simulink model "EcoSIM3_P2_C2_WIP"  (R2014b)
settings: Solver=ode1  SolverMode=SingleTasking  StartTime=0.0  StopTime=4  FixedStep=0.01  RelTol=1e-3
PostLoadFcn:
  | %, if any(exist('dsrtsu_mdlpostloadfcn', 'file') == [2, 3, 6]), try dsrtsu_mdlpostloadfcn('Execute', bdroot); catch fprintf('Error in PostLoadFcn (dsrtsu_mdlpostloadfcn) for model "%s":\n %s\n', bdroot, lasterr); end, end,
InitFcn:
  | tic
  | %Startup_EcoSIM
undefined symbols (not defined in the file or in its folder): canChannel, Controls, DriveCycles, Driver, EM_EFF_MAP, EM_PwrLoss_MAP, EngPwr, EngSpd, EngTrq, Glbl, Overwritten_Mode, Plants, Power, sigbuilder_block, Torque, Trialmap, Veh_Dynamics
libraries: simulink x135, canmsglib x113, fl_lib x104, canlib x89, nesl_utility x56, sdl_lib x29, dspsigops x6, dspswit3 x5, dspstat3 x2, commnoisgen2 x1, dspfdesign x1
(part 12 of 21)

== system EcoSIM3_P2_C2_WIP/Powertrain/Soft_ECUs_IO/VNT Vector/CANTx/EM ==
  EM : Inport
  CAN Transmit1 : canlib/CAN Transmit  BlockHandle=11751.0004  DeviceMenu=Vector Virtual 1 (Channel 2)  Device=Vector Virtual 1 (Channel 2)  ObjConstructor=canChannel('Vector', 'Virtual 1', 2)  EnablePeriodicTransmit=off  MessagePeriod=1.000
  M160_Temperature_Set_1 : Subsystem
  M161_Temperature_Set_2 : Subsystem
  M162_Temperature_Set_3 : Subsystem
  M165_Motor_Position_Info : Subsystem
  M170_Internal_States : Subsystem
  M171_Fault_Codes : Subsystem
  M172_Torque_And_Timer_Info : Subsystem
  Mux : Mux  Inputs=7
  wires:
  EM/1 -> M160_Temperature_Set_1/1(EM), M161_Temperature_Set_2/1(EM), M162_Temperature_Set_3/1(EM), M170_Internal_States/1(EM), M172_Torque_And_Timer_Info/1(EM), M165_Motor_Position_Info/1(EM), M171_Fault_Codes/1(EM)
  M165_Motor_Position_Info/1(Out1) -> Mux/1
  M172_Torque_And_Timer_Info/1(Out1) -> Mux/2
  M170_Internal_States/1(Out1) -> Mux/3
  M171_Fault_Codes/1(Out1) -> Mux/4
  M160_Temperature_Set_1/1(Out1) -> Mux/5
  M161_Temperature_Set_2/1(Out1) -> Mux/6
  M162_Temperature_Set_3/1(Out1) -> Mux/7
  Mux/1 -> CAN Transmit1/1

== system EcoSIM3_P2_C2_WIP/Powertrain/Soft_ECUs_IO/VNT Vector/CANTx/ESS ==
  ESS : Inport
  BCM_Data : Subsystem
  BCM_Limits : Subsystem
  BCM_Status : Subsystem
  wires:
  ESS/1 -> BCM_Data/1(ESS), BCM_Status/1(ESS), BCM_Limits/1(ESS)

== system EcoSIM3_P2_C2_WIP/Powertrain/Soft_ECUs_IO/VNT Vector/CANTx/Engine ==
  ICE : Inport
  Bus Selector1 : BusSelector  OutputSignals=ICE_Torque.ICE_Torque_Cmd_Nm
  CAN Pack : canmsglib/CAN Pack  CANdbFile=C:\Users\EcoCAR_HIL\Documents\Khanna\EcoSIM3_P1_0_PHEV_TCU\Final_DBC\Engine_Transmission_BAS.dbc  MsgList=ECO_Engine_MSG104  MsgName=ECO_Engine_MSG104  MsgIDType=Standard (11-bit identifier)  MsgIdentifier=104  MsgLength=2  SignalInfo=ICE_Torque_Cmd_Nm$9$15$2$2$1$0$1.000000e-02$0$0$3.276700e+02$#  NSignals=1  StartBits=str2num('[int32(9)]')  SignalSizes=str2num('[int32(15)]')  ByteOrders=str2num('[int32(2)]')  DataTypes=str2num('[int32(2)]')  MultiplexTypes=str2num('[int32(1)]')  MultiplexValues=str2num('[double(0)]')  Factors=str2num('[double(1.000000e-02)]')  Offsets=str2num('[double(0)]')  Minimums=str2num('[double(0)]')  Maximums=str2num('[double(3.276700e+02)]')  Remote=off
      settings: DataFormat=CANdb specified signals
  CAN Transmit : canlib/CAN Transmit  BlockHandle=12006.0001  DeviceMenu=Vector Virtual 1 (Channel 1)  Device=Vector Virtual 1 (Channel 1)  ObjConstructor=canChannel('Vector', 'Virtual 1', 1)  EnablePeriodicTransmit=off  MessagePeriod=1.000
  Rate Transition4 : RateTransition
  wires:
  CAN Pack/1 -> CAN Transmit/1
  Bus Selector1/1 -> Rate Transition4/1  "<ICE_Torque_Cmd_Nm>"
  ICE/1 -> Bus Selector1/1
  Rate Transition4/1 -> CAN Pack/1

== system EcoSIM3_P2_C2_WIP/Powertrain/Soft_ECUs_IO/VNT Vector/CANTx/GMLAN ==
  Driver : Inport
  CAN Transmit2 : canlib/CAN Transmit  BlockHandle=12014.0001  DeviceMenu=Vector Virtual 1 (Channel 1)  Device=Vector Virtual 1 (Channel 1)  ObjConstructor=canChannel('Vector', 'Virtual 1', 1)  EnablePeriodicTransmit=off  MessagePeriod=1.000
  Mux : Mux  Inputs=5
  PPEI_Brake_Apply_Status : Subsystem
  PPEI_Driven_Whl_Rotational_Stat : Subsystem
  PPEI_NonDrivn_Whl_Rotational_Stat : Subsystem
  PPEI_Platform_General_Status : Subsystem
  PPEI_Vehicle_Speed_and_Distance : Subsystem
  wires:
  Driver/1 -> PPEI_Vehicle_Speed_and_Distance/1(GM), PPEI_NonDrivn_Whl_Rotational_Stat/1(GM), PPEI_Driven_Whl_Rotational_Stat/1(GM), PPEI_Platform_General_Status/1(GM), PPEI_Brake_Apply_Status/1(GM)
  PPEI_Platform_General_Status/1(Out1) -> Mux/1
  PPEI_Brake_Apply_Status/1(Out1) -> Mux/2
  PPEI_Vehicle_Speed_and_Distance/1(Out1) -> Mux/3
  PPEI_Driven_Whl_Rotational_Stat/1(Out1) -> Mux/4
  PPEI_NonDrivn_Whl_Rotational_Stat/1(Out1) -> Mux/5
  Mux/1 -> CAN Transmit2/1

== system EcoSIM3_P2_C2_WIP/Powertrain/Soft_ECUs_IO/VNT Vector/ElectricalRx/BAS_Relay ==
  In1 : Inport
  Constant6 : Constant
  Constant7 : Constant  Value=0
  Relay3 : Switch  Criteria=u2 > Threshold  Threshold=0.5
  Out1 : Outport
  wires:
  In1/1 -> Relay3/2
  Constant7/1 -> Relay3/3
  Relay3/1 -> Out1/1  "BAS_Powerup"
  Constant6/1 -> Relay3/1

== system EcoSIM3_P2_C2_WIP/Powertrain/Soft_ECUs_IO/VNT Vector/ElectricalRx/BMS Electrical ==
  In1 : Inport
  In2 : Inport  Port=2
  In3 : Inport  Port=3
  Bus Creator8 : BusCreator  Inputs=3
  Constant : Constant
  Constant1 : Constant  Value=0
  Constant2 : Constant
  Constant3 : Constant  Value=0
  Relay : Switch  Criteria=u2 > Threshold  Threshold=0.5
  Relay1 : Switch  Criteria=u2 > Threshold  Threshold=0.5
  Out1 : Outport
  wires:
  In2/1 -> Relay/2
  Constant/1 -> Relay/1
  In1/1 -> Bus Creator8/1
  Constant1/1 -> Relay/3
  Bus Creator8/1 -> Out1/1  "BCM_Electrical"
  Relay/1 -> Bus Creator8/2  "BMS_Powerup"
  Constant2/1 -> Relay1/1
  Constant3/1 -> Relay1/3
  In3/1 -> Relay1/2
  Relay1/1 -> Bus Creator8/3  "veh_wake"

== system EcoSIM3_P2_C2_WIP/Powertrain/Soft_ECUs_IO/VNT Vector/ElectricalRx/EM_Relay ==
  In1 : Inport
  Constant2 : Constant
  Constant3 : Constant  Value=0
  Relay1 : Switch  Criteria=u2 > Threshold  Threshold=0.5
  Out1 : Outport
  wires:
  In1/1 -> Relay1/2
  Constant3/1 -> Relay1/3
  Constant2/1 -> Relay1/1
  Relay1/1 -> Out1/1  "EM_Powerup"

== system EcoSIM3_P2_C2_WIP/Powertrain/Soft_ECUs_IO/VNT Vector/ElectricalRx/Engine_Relay ==
  In1 : Inport
  Constant4 : Constant
  Constant5 : Constant  Value=0
  Relay2 : Switch  Criteria=u2 > Threshold  Threshold=0.5
  Out1 : Outport
  wires:
  In1/1 -> Relay2/2
  Constant4/1 -> Relay2/1
  Constant5/1 -> Relay2/3
  Relay2/1 -> Out1/1  "ICE_Powerup"

== system EcoSIM3_P2_C2_WIP/Powertrain/Soft_ECUs_IO/VNT Vector/ElectricalRx/Mastershift ==
  MShift : Inport
  Bus Creator : BusCreator  Inputs=3
  Bus Selector : BusSelector  OutputSignals=Upshift_Sw,Downshift_Sw,Clutch_Sw
  Out1 : Outport
  wires:
  MShift/1 -> Bus Selector/1
  Bus Selector/1 -> Bus Creator/1  "<Upshift_Sw>"
  Bus Selector/3 -> Bus Creator/3  "<Clutch_Sw>"
  Bus Selector/2 -> Bus Creator/2  "<Downshift_Sw>"
  Bus Creator/1 -> Out1/1  "Mastershift_Electrical"

== system EcoSIM3_P2_C2_WIP/RTI Data/RTI Data Store/RTI Data Store/RTI Data Store/RTI Data Store ==

== system EcoSIM3_P2_C2_WIP/Supervisory Controller/Functional Safety1/Functional Safety Algorithm/Fault Detection (Team Developed)/Accelerator Pedal Faults ==
  In1 : Inport
  Ground : Ground
  Terminator : Terminator
  Out1 : Outport
  wires:
  In1/1 -> Terminator/1
  Ground/1 -> Out1/1

== system EcoSIM3_P2_C2_WIP/Supervisory Controller/Functional Safety1/Functional Safety Algorithm/Fault Detection (Team Developed)/Brake Pedal Faults ==
  In1 : Inport
  Ground : Ground
  Terminator : Terminator
  Out1 : Outport
  wires:
  In1/1 -> Terminator/1
  Ground/1 -> Out1/1

== system EcoSIM3_P2_C2_WIP/Supervisory Controller/Functional Safety1/Functional Safety Algorithm/Fault Detection (Team Developed)/Drivetrain Faults ==
  In1 : Inport
  Ground : Ground
  Terminator : Terminator
  Out1 : Outport
  wires:
  In1/1 -> Terminator/1
  Ground/1 -> Out1/1

== system EcoSIM3_P2_C2_WIP/Supervisory Controller/Functional Safety1/Functional Safety Algorithm/Fault Detection (Team Developed)/Parking Brake Faults ==
  In1 : Inport
  Ground : Ground
  Terminator : Terminator
  Out1 : Outport
  wires:
  In1/1 -> Terminator/1
  Ground/1 -> Out1/1

== system EcoSIM3_P2_C2_WIP/Supervisory Controller/Functional Safety1/Functional Safety Algorithm/Fault Detection (Team Developed)/Torque Security Faults ==
  Torque Requests : Inport
  ECU/Sensor Signals : Inport  Port=2
  Torque Comparisons : Subsystem
  Torque Estimation : Subsystem
  Vehicle Mass Estimation : Subsystem  Commented=on
  Faults : Outport
  wires:
  ECU/Sensor Signals/1 -> Torque Comparisons/2(Torque Feedbacks), Torque Estimation/2(ECU/Sensor Signals), Vehicle Mass Estimation/1(In1)
  Torque Requests/1 -> Torque Comparisons/3(Torque Requests)
  Vehicle Mass Estimation/1(Veh Mass Est) -> Torque Estimation/1(Veh Mass Est)
  Torque Comparisons/1(Faults) -> Faults/1
  Torque Estimation/1(Torque_Estimates) -> Torque Comparisons/1(Torque Estimates)

== system EcoSIM3_P2_C2_WIP/Supervisory Controller/Mode Operation/Engine Only /Subsystem/Engine Torque Calc ==
  note: This will be torque at the wheels
  note: Torque requested at Engine
  Gear : Inport
  Vehicle Speed : Inport  Port=2
  Torque Request : Inport  Port=3
  Max Torque Calculation : Subsystem
  Min Torque : Constant  Value=0
  Saturation Dynamic : simulink/Discontinuities/Saturation Dynamic  OutMin=[]  OutMax=[]  OutDataTypeStr=Inherit: Same as second input  OutDataType=fixdt(1, 16)  OutScaling=2^-10  DoSatur=off
  Speed Calculations : Subsystem
  Eng_T_Opt : Outport
  wires:
  Max Torque Calculation/1("Engine Torque ") -> Saturation Dynamic/1
  Gear/1 -> Max Torque Calculation/2(Gear), Speed Calculations/2(Gear Current)
  Speed Calculations/1(Engine Speed) -> Max Torque Calculation/1(In1)
  Vehicle Speed/1 -> Speed Calculations/1("Vehicle Speed m/s ")
  Min Torque/1 -> Saturation Dynamic/3
  Saturation Dynamic/1 -> Eng_T_Opt/1  "Need some kind  of rate limiter"
  Torque Request/1 -> Saturation Dynamic/2

== system EcoSIM3_P2_C2_WIP/Supervisory Controller/Mode Operation/Engine Only /Subsystem/Gear Shift Requested 1 ==
  "Current Gear " : Inport
  Vehicle_Speed [m/s] : Inport  Port=2
  ICE_Torque_CMD [Nm] : Inport  Port=3
  Data Type Conversion : DataTypeConversion  OutMin=[0]  OutMax=[1]  OutDataTypeStr=double
  Diff_GR : Gain  Gain=Plants.Rear_Diff.Diff_ratio
  Memory : Memory  InheritSampleTime=on
  Multiply : Product  Inputs=**
  Relational Operator : RelationalOperator  Operator=~=  OutDataTypeStr=boolean
  Switch : Switch  Threshold=1
  Trans GR : Lookup  InputValues=Plants.Trans.Mdl.Plant.Gear_cmd  Table=Plants.Trans.Mdl.Plant.GR  LookUpMeth=Use Input Nearest
  optimal gear map : Lookup_n-D  BreakpointsForDimension1=Controls.Trans.shiftmap.vehspd  BreakpointsForDimension2=Controls.Trans.shiftmap.whltrq  Table=Controls.Trans.shiftmap.gear  InterpMethod=Nearest  InternalRulePriority=Speed  RndMeth=Simplest  InputSameDT=on
  "Shift Requested " : Outport
  "Gear Requested " : Outport  Port=2
  wires:
  Relational Operator/1 -> Data Type Conversion/1, Switch/2
  Switch/1 -> "Gear Requested "/1  "Gear Requested"
  "Current Gear "/1 -> Switch/3, Relational Operator/1
  Data Type Conversion/1 -> "Shift Requested "/1  "Shift Requested"
  ICE_Torque_CMD [Nm]/1 -> Multiply/1
  Memory/1 -> Trans GR/1
  Trans GR/1 -> Multiply/2
  Diff_GR/1 -> optimal gear map/2
  optimal gear map/1 -> Relational Operator/2, Switch/1, Memory/1  "Gear_Request"
  Vehicle_Speed [m/s]/1 -> optimal gear map/1
  Multiply/1 -> Diff_GR/1

== system EcoSIM3_P2_C2_WIP/Supervisory Controller/Mode Operation/Engine Start /BAS_Signals1/Subsystem ==
  BAS_Desired_Speed [rad/s] : Inport
  BAS_Speed [rad/s] : Inport  Port=2
  Compare To Zero1 : simulink/Logic and Bit Operations/Compare To Zero  relop===  OutDataTypeStr=boolean  ZeroCross=off
  Delay : Subsystem
  I : Constant  Value=0.2
  Integrator1 : Integrator  ExternalReset=level
  P : Constant  Value=40
  Product3 : Product  RndMeth=Zero
  Product4 : Product  RndMeth=Zero
  Scope : Scope
      settings: SaveName=ScopeData32
  Sum3 : Sum  Inputs=|-+  SaturateOnIntegerOverflow=on  InputSameDT=on  OutDataTypeStr=Inherit: Same as first input
  Sum4 : Sum  SaturateOnIntegerOverflow=on  InputSameDT=on  OutDataTypeStr=Inherit: Same as first input
  Sum5 : Sum  Inputs=|+-  SaturateOnIntegerOverflow=on  InputSameDT=on  OutDataTypeStr=Inherit: Same as first input
  BAS_Torque_Request : Outport
  wires:
  BAS_Speed [rad/s]/1 -> Sum3/1, Compare To Zero1/1, Sum5/2
  Compare To Zero1/1 -> Integrator1/2
  Product3/1 -> Sum4/2
  Product4/1 -> Sum4/1
  Integrator1/1 -> Product3/1
  Sum3/1 -> Integrator1/1
  P/1 -> Product4/1
  BAS_Desired_Speed [rad/s]/1 -> Delay/1(BAS_Speed_Rad_per_sec), Sum5/1
  Delay/1(Pre_BAS_Speed_Rad_per_sec) -> Sum3/2
  Sum5/1 -> Product4/2
  I/1 -> Product3/2
  Sum4/1 -> Scope/1, BAS_Torque_Request/1

== system EcoSIM3_P2_C2_WIP/Supervisory Controller/Mode Operation/Limited EV/ICE_torque/Engine Messages1 ==
  Torque : Inport
  Bus Creator2 : BusCreator  Inputs=3
  Constant2 : Constant
  Constant3 : Constant
  Gain : Gain
  ICE_Request : Outport
  wires:
  Gain/1 -> Bus Creator2/1  "ICE_Torque_Request_Nm"
  Constant2/1 -> Bus Creator2/2  "Engine_On"
  Constant3/1 -> Bus Creator2/3  "Engine_Run"
  Bus Creator2/1 -> ICE_Request/1  "ICE_Request"
  Torque/1 -> Gain/1

== system EcoSIM3_P2_C2_WIP/Supervisory Controller/Mode Operation/Limited EV/ICE_torque/ICE Torque Request & Gear Selection  ==
  note: Changing input signal affects rate limiter in engine softecu
  note: Should this be driver torque request or engine actual torque command?
  Vehicle_Speed [m/s] : Inport
  ICE_Torque_CMD [Nm] : Inport  Port=2
  ICE_Torque_Request : Inport  Port=3
  Diff_GR : Gain  Gain=Plants.Rear_Diff.Diff_ratio
  Diff_GR1 : Gain  Gain=1/Plants.Rear_Diff.Diff_ratio
  Divide : Product  Inputs=/*
  Memory : Memory  InheritSampleTime=on
  Multiply : Product  Inputs=**
  Trans GR : Lookup  InputValues=Plants.Trans.Mdl.Plant.Gear_cmd  Table=Plants.Trans.Mdl.Plant.GR  LookUpMeth=Use Input Nearest
  Trial gear map : Lookup_n-D  Commented=on  BreakpointsForDimension1=Trialmap.Vehspdkph  BreakpointsForDimension2=Trialmap.AcPedalPosn  Table=Trialmap.Gear  InterpMethod=Nearest  InternalRulePriority=Speed  RndMeth=Simplest  InputSameDT=on
  optimal gear map : Lookup_n-D  BreakpointsForDimension1=Controls.Trans.shiftmap.vehspd  BreakpointsForDimension2=Controls.Trans.shiftmap.whltrq  Table=Controls.Trans.shiftmap.gear  InterpMethod=Nearest  InternalRulePriority=Speed  RndMeth=Simplest  InputSameDT=on
  ICE_Torque_Request [Nm] : Outport
  Gear_Request[-] : Outport  Port=2
  wires:
  Multiply/1 -> Diff_GR/1
  optimal gear map/1 -> Gear_Request[-]/1, Memory/1  "Gear_Request"
  Trans GR/1 -> Divide/1, Multiply/2
  Memory/1 -> Trans GR/1
  Vehicle_Speed [m/s]/1 -> optimal gear map/1
  Diff_GR/1 -> optimal gear map/2
  ICE_Torque_CMD [Nm]/1 -> Multiply/1
  Divide/1 -> Diff_GR1/1
  Diff_GR1/1 -> ICE_Torque_Request [Nm]/1
  ICE_Torque_Request/1 -> Divide/2

== system EcoSIM3_P2_C2_WIP/Supervisory Controller/Mode Operation/Limited EV/ICE_torque/Trans Clutch Messages ==
  Gear Request : Inport
  CAN : Inport  Port=2
  Bus Creator6 : BusCreator  Inputs=2
  Bus Selector : BusSelector  OutputSignals=BAS_Transmit.BAS_CAN_Out.Status_1.BAS_Speed_rad_per_s,Vehicle_speed.Vehicle_Speed_meter_per_s,GM_Transmit.GMLAN_CAN_Out.PPEI_Brake_Apply_Status.BrkPdlPos
  Compare To Constant1 : simulink/Logic and Bit Operations/Compare To Constant  relop=>  const=1  OutDataTypeStr=boolean
  Compare To Constant2 : simulink/Logic and Bit Operations/Compare To Constant  relop=<=  const=2  OutDataTypeStr=boolean
  Constant : Constant  Value=0.9774*169.646
  Constant1 : Constant  Commented=on
  Constant5 : Constant  Value=197.920
  Data Type Conversion : DataTypeConversion  OutMin=[0]  OutMax=[1]  OutDataTypeStr=double
  Gain : Gain  Gain=0.01
  GentleClutchRelease : Stateflow chart  TreatAsAtomicUnit=on
  IC : InitialCondition  Value=0
  Logical Operator : Logic  Operator=NOT  AllPortsSameDT=off  OutDataTypeStr=boolean
  Logical Operator1 : Logic  AllPortsSameDT=off  OutDataTypeStr=boolean
  Rate Limiter : RateLimiter  RisingSlewLimit=inf  SampleTimeMode=inherited
  Terminator : Terminator
  Trans_Receive : Outport
  wires:
  IC/1 -> GentleClutchRelease/2(Clutch_Request)  "Shift_Request"
  Rate Limiter/1 -> Terminator/1, Bus Creator6/1  "Shift_Request"
  CAN/1 -> Bus Selector/1
  Bus Creator6/1 -> Trans_Receive/1  "Trans_Receive"
  Compare To Constant1/1 -> Logical Operator1/2
  Gear Request/1 -> Bus Creator6/2
  Logical Operator/1 -> Data Type Conversion/1
  Logical Operator1/1 -> Logical Operator/1
  Bus Selector/3 -> Compare To Constant1/1  "<BrkPdlPos>"
  Compare To Constant2/1 -> Logical Operator1/1
  Constant/1 -> GentleClutchRelease/3(Lower_Clutch_Speed)
  Constant5/1 -> GentleClutchRelease/4(Upper_Clutch_Speed)
  Bus Selector/1 -> GentleClutchRelease/1(BAS_Speed)  "<BAS_Speed_rad_per_s>"
  GentleClutchRelease/1(Shift_Request) -> Gain/1  "Clutch_Request_Percent"
  Bus Selector/2 -> Compare To Constant2/1  "<Vehicle_Speed_meter_per_s>"
  Data Type Conversion/1 -> IC/1  "Shift_Request"
  Gain/1 -> Rate Limiter/1

== system EcoSIM3_P2_C2_WIP/Supervisory Controller/Mode Operation/Series/Series Torque Determination /SOC Control ==
  Battery SOC : Inport
  SOC Target : Inport  Port=2
  Terminator : Terminator
  Power Request : Outport
  wires:
  Battery SOC/1 -> Power Request/1
  SOC Target/1 -> Terminator/1

== system EcoSIM3_P2_C2_WIP/Supervisory Controller/Mode Operation/Series1/BAS_Signals/Enabled Subsystem1 ==
  BAS_Speed [rad/s] : Inport
  Desired_Speed : Inport  Port=2
  Compare To Zero1 : simulink/Logic and Bit Operations/Compare To Zero  relop===  OutDataTypeStr=boolean  ZeroCross=off
  Delay : Subsystem
  I : Constant  Value=0.1
  Integrator1 : Integrator  ExternalReset=level
  P : Constant  Value=10
  Product3 : Product  RndMeth=Zero
  Product4 : Product  RndMeth=Zero
  Sum3 : Sum  Inputs=|-+  SaturateOnIntegerOverflow=on  InputSameDT=on  OutDataTypeStr=Inherit: Same as first input
  Sum4 : Sum  SaturateOnIntegerOverflow=on  InputSameDT=on  OutDataTypeStr=Inherit: Same as first input
  Sum5 : Sum  Inputs=|+-  SaturateOnIntegerOverflow=on  InputSameDT=on  OutDataTypeStr=Inherit: Same as first input
  "Torque Command " : Outport
  wires:
  Sum4/1 -> "Torque Command "/1
  BAS_Speed [rad/s]/1 -> Sum3/1, Compare To Zero1/1, Sum5/2
  Compare To Zero1/1 -> Integrator1/2
  Product3/1 -> Sum4/2
  Product4/1 -> Sum4/1
  Integrator1/1 -> Product3/1
  Sum3/1 -> Integrator1/1
  P/1 -> Product4/1
  Desired_Speed/1 -> Delay/1(BAS_Speed_Rad_per_sec), Sum5/1
  Delay/1(Pre_BAS_Speed_Rad_per_sec) -> Sum3/2
  Sum5/1 -> Product4/2
  I/1 -> Product3/2

== system EcoSIM3_P2_C2_WIP/Supervisory Controller/PRNDL/Reverse/Ensure Desired Rotation Direction/TOGGLE ==
  Enable : EnablePort
  Add : Sum
  Constant : Constant
  Constant1 : Constant  Value=0
  Tapped Delay : simulink/Discrete/Tapped Delay  vinit=0.0  samptime=.5  NumDelays=1  DelayOrder=Oldest  includeCurrent=off
  Out1 : Outport
  wires:
  Constant1/1 -> Add/2
  Tapped Delay/1 -> Add/1
  Add/1 -> Out1/1
  Constant/1 -> Tapped Delay/1

== system EcoSIM3_P2_C2_WIP/Supervisory Controller/Supervisory_IO/VNT Kvaser/CAN Rx/BAS ==
  Bus Creator : BusCreator  Inputs=2
  Bus Creator1 : BusCreator  Inputs=2
  Bus Creator2 : BusCreator  Inputs=3
  CAN Receive5 : canlib/CAN Receive  BlockHandle=3010.0022  DeviceMenu=Kvaser Virtual 1 (Channel 1)  Device=Kvaser Virtual 1 (Channel 1)  ObjConstructor=canChannel('Kvaser', 'Virtual 1', 1)  EnableStandardIDsFilter=off  StandardIDs=99  EnableExtendedIDsFilter=off  ExtendedIDs=0  SampleTime=0.01  MsgsPerTimestep=1  StdIDsCombo=Allow only  ExtIDsCombo=Block all  InternalFilterUpdateStatus=on
  CAN Unpack5 : canmsglib/CAN Unpack  CANdbFile=C:\Users\EcoCAR_HIL\Documents\Khanna\EcoSIM3_P1_0_PHEV_TCU\Final_DBC\Engine_Transmission_BAS.dbc  MsgList=ECO_BAS_Status_MSG099  MsgName=ECO_BAS_Status_MSG099  MsgIDType=Standard (11-bit identifier)  MsgIdentifier=99  MsgLength=5  SignalInfo=BAS_Fault_Status$36$1$2$2$1$0$1$0$0$1$#BAS_Speed_rad_per_s$8$16$2$1$1$0$1.000000e-01$0$-3.276800e+03$3.276700e+03$#BAS_Status_Mode$37$1$2$2$1$0$1$0$0$1$#BAS_Torque_Command_Nm$25$15$2$1$1$0$1.000000e-02$0$-1.638400e+02$1.638300e+02$#Fault_U$24$1$2$2$1$0$1$0$0$1$#Fault_V$39$1$2$2$1$0$1$0$0$1$#Fault_W$38$1$2$2$1$0$1$0$0$1$#  NSignals=7  IDPort=off  TimestampPort=off  ErrorPort=off  RemotePort=off  LengthPort=off  StatusPort=off  StartBits=str2num('[int32(36);int32(8);int32(37);int32(25);int32(24);int32(39);int32(38)]')  SignalSizes=str2num('[int32(1);int32(16);int32(1);int32(15);int32(1);int32(1);int32(1)]')  ByteOrders=str2num('[int32(2);int32(2);int32(2);int32(2);int32(2);int32(2);int32(2)]')  DataTypes=str2num('[int32(2);int32(1);int32(2);int32(1);int32(2);int32(2);int32(2)]')  MultiplexTypes=str2num('[int32(1);int32(1);int32(1);int32(1);int32(1);int32(1);int32(1)]')  MultiplexValues=str2num('[double(0);double(0);double(0);double(0);double(0);double(0);double(0)]')  Factors=str2num('[double(1);double(1.000000e-01);double(1);double(1.000000e-02);double(1);double(1);double(1)]')  Offsets=str2num('[double(0);double(0);double(0);double(0);double(0);double(0);double(0)]')  Minimums=str2num('[double(0);double(-3.276800e+03);double(0);double(-1.638400e+02);double(0);double(0);double(0)]')  Maximums=str2num('[double(1);double(3.276700e+03);double(1);double(1.638300e+02);double(1);double(1);double(1)]')
      settings: DataFormat=CANdb specified signals
  Terminator : Terminator
  Terminator1 : Terminator
  Terminator27 : Terminator
  BAS : Outport
  wires:
  CAN Receive5/2 -> CAN Unpack5/1
  CAN Receive5/1 -> Terminator27/1
  CAN Unpack5/7 -> Bus Creator2/3  "Fault_W"
  CAN Unpack5/6 -> Bus Creator2/2  "Fault_V"
  CAN Unpack5/5 -> Bus Creator2/1  "Fault_U"
  CAN Unpack5/4 -> Bus Creator1/2  "BAS_Torque_Out_Nm"
  CAN Unpack5/3 -> Terminator1/1  "BAS_Status_Mode"
  CAN Unpack5/2 -> Bus Creator1/1  "BAS_Speed_rad_per_s"
  CAN Unpack5/1 -> Terminator/1  "BAS_Fault_Status"
  Bus Creator1/1 -> Bus Creator/1  "Status_1"
  Bus Creator2/1 -> Bus Creator/2  "Status_2"
  Bus Creator/1 -> BAS/1  "BAS_CAN_Out"

== system EcoSIM3_P2_C2_WIP/Supervisory Controller/Supervisory_IO/VNT Kvaser/CAN Rx/Clutch Transmission ==
  Bus Creator : BusCreator  Inputs=1
  Bus Creator1 : BusCreator  Inputs=1
  CAN Receive3 : canlib/CAN Receive  BlockHandle=7374.0027  DeviceMenu=Kvaser Virtual 1 (Channel 1)  Device=Kvaser Virtual 1 (Channel 1)  ObjConstructor=canChannel('Kvaser', 'Virtual 1', 1)  EnableStandardIDsFilter=off  StandardIDs=106  EnableExtendedIDsFilter=off  ExtendedIDs=0  SampleTime=0.01  MsgsPerTimestep=1  StdIDsCombo=Allow only  ExtIDsCombo=Block all  InternalFilterUpdateStatus=on
  CAN Unpack3 : canmsglib/CAN Unpack  CANdbFile=C:\Users\EcoCAR_HIL\Documents\Khanna\EcoSIM3_P1_0_PHEV_TCU\Final_DBC\Engine_Transmission_BAS.dbc  MsgList=ECO_Trans_Status_MSG106  MsgName=ECO_Trans_Status_MSG106  MsgIDType=Standard (11-bit identifier)  MsgIdentifier=106  MsgLength=1  SignalInfo=Actual_Gear$1$3$2$2$1$0$1$0$0$7$#Clutch_Sw$7$1$2$2$1$0$1$0$0$1$#TCM_Gear$4$3$2$2$1$0$1$0$0$7$#  NSignals=3  IDPort=off  TimestampPort=off  ErrorPort=off  RemotePort=off  LengthPort=off  StatusPort=off  StartBits=str2num('[int32(1);int32(7);int32(4)]')  SignalSizes=str2num('[int32(3);int32(1);int32(3)]')  ByteOrders=str2num('[int32(2);int32(2);int32(2)]')  DataTypes=str2num('[int32(2);int32(2);int32(2)]')  MultiplexTypes=str2num('[int32(1);int32(1);int32(1)]')  MultiplexValues=str2num('[double(0);double(0);double(0)]')  Factors=str2num('[double(1);double(1);double(1)]')  Offsets=str2num('[double(0);double(0);double(0)]')  Minimums=str2num('[double(0);double(0);double(0)]')  Maximums=str2num('[double(7);double(1);double(7)]')
      settings: DataFormat=CANdb specified signals
  Terminator12 : Terminator
  Terminator28 : Terminator
  Terminator29 : Terminator
  Trans : Outport
  wires:
  CAN Receive3/1 -> Terminator12/1
  CAN Unpack3/1 -> Bus Creator1/1  "Actual_Gear"
  CAN Receive3/2 -> CAN Unpack3/1
  CAN Unpack3/2 -> Terminator28/1  "Clutch_Sw"
  CAN Unpack3/3 -> Terminator29/1  "TCM_Gear"
  Bus Creator1/1 -> Bus Creator/1  "Message_1"
  Bus Creator/1 -> Trans/1  "Clutch_Transmission_CAN_Out"

== system EcoSIM3_P2_C2_WIP/Supervisory Controller/Supervisory_IO/VNT Kvaser/CAN Rx/ESS ==
  Bus Creator : BusCreator  Inputs=3
  Bus Creator1 : BusCreator  Inputs=11
  Bus Creator2 : BusCreator  Inputs=3
  Bus Creator3 : BusCreator  Inputs=2
  CAN Receive1 : canlib/CAN Receive  BlockHandle=7392.0026  DeviceMenu=Kvaser Virtual 1 (Channel 1)  Device=Kvaser Virtual 1 (Channel 1)  ObjConstructor=canChannel('Kvaser', 'Virtual 1', 1)  EnableStandardIDsFilter=off  StandardIDs=1072  EnableExtendedIDsFilter=off  ExtendedIDs=0  SampleTime=0.01  MsgsPerTimestep=1  StdIDsCombo=Allow only  ExtIDsCombo=Block all  InternalFilterUpdateStatus=on
  CAN Receive2 : canlib/CAN Receive  BlockHandle=7393.0023  DeviceMenu=Kvaser Virtual 1 (Channel 1)  Device=Kvaser Virtual 1 (Channel 1)  ObjConstructor=canChannel('Kvaser', 'Virtual 1', 1)  EnableStandardIDsFilter=off  StandardIDs=1040  EnableExtendedIDsFilter=off  ExtendedIDs=0  SampleTime=0.01  MsgsPerTimestep=1  StdIDsCombo=Allow only  ExtIDsCombo=Block all  InternalFilterUpdateStatus=on
  CAN Receive3 : canlib/CAN Receive  BlockHandle=7394.0023  DeviceMenu=Kvaser Virtual 1 (Channel 1)  Device=Kvaser Virtual 1 (Channel 1)  ObjConstructor=canChannel('Kvaser', 'Virtual 1', 1)  EnableStandardIDsFilter=off  StandardIDs=1056  EnableExtendedIDsFilter=off  ExtendedIDs=0  SampleTime=0.01  MsgsPerTimestep=1  StdIDsCombo=Allow only  ExtIDsCombo=Block all  InternalFilterUpdateStatus=on
  CAN Unpack1 : canmsglib/CAN Unpack  CANdbFile=C:\Users\EcoCAR_HIL\Documents\Khanna\EcoSIM3_P1_0_PHEV_TCU\Final_DBC\BCM_VehBus_Std.dbc  MsgList=BCM_Limits  MsgName=BCM_Limits  MsgIDType=Standard (11-bit identifier)  MsgIdentifier=1056  MsgLength=8  SignalInfo=bcm_cell_overvolt$55$1$2$2$1$0$1$0$0$1$#bcm_cell_undervolt$54$1$2$2$1$0$1$0$0$1$#bcm_chg_buf$32$8$2$2$1$0$5.000000e-01$0$0$100$#bcm_chg_max$16$12$2$2$1$0$2.500000e-01$0$0$1000$#bcm_dis_buf$24$8$2$2$1$0$5.000000e-01$0$0$100$#bcm_dis_max$12$12$2$2$1$0$2.500000e-01$0$0$1000$#bcm_t_coolant$40$8$2$2$1$0$5.000000e-01$-40$-40$85$#  NSignals=7  IDPort=off  TimestampPort=off  ErrorPort=off  RemotePort=off  LengthPort=off  StatusPort=off  StartBits=str2num('[int32(55);int32(54);int32(32);int32(16);int32(24);int32(12);int32(40)]')  SignalSizes=str2num('[int32(1);int32(1);int32(8);int32(12);int32(8);int32(12);int32(8)]')  ByteOrders=str2num('[int32(2);int32(2);int32(2);int32(2);int32(2);int32(2);int32(2)]')  DataTypes=str2num('[int32(2);int32(2);int32(2);int32(2);int32(2);int32(2);int32(2)]')  MultiplexTypes=str2num('[int32(1);int32(1);int32(1);int32(1);int32(1);int32(1);int32(1)]')  MultiplexValues=str2num('[double(0);double(0);double(0);double(0);double(0);double(0);double(0)]')  Factors=str2num('[double(1);double(1);double(5.000000e-01);double(2.500000e-01);double(5.000000e-01);double(2.500000e-01);double(5.000000e-01)]')  Offsets=str2num('[double(0);double(0);double(0);double(0);double(0);double(0);double(-40)]')  Minimums=str2num('[double(0);double(0);double(0);double(0);double(0);double(0);double(-40)]')  Maximums=str2num('[double(1);double(1);double(100);double(1000);double(100);double(1000);double(85)]')
      settings: DataFormat=CANdb specified signals
  CAN Unpack2 : canmsglib/CAN Unpack  CANdbFile=C:\Users\EcoCAR_HIL\Documents\Khanna\EcoSIM3_P1_0_PHEV_TCU\Final_DBC\BCM_VehBus_Std.dbc  MsgList=BCM_Status  MsgName=BCM_Status  MsgIDType=Standard (11-bit identifier)  MsgIdentifier=1040  MsgLength=8  SignalInfo=bcm_alarm$14$2$2$2$1$0$1$0$0$3$#bcm_chg_done$52$1$2$2$1$0$1$0$0$1$#bcm_chgc_stat$6$2$2$2$1$0$1$0$0$2$#bcm_cool_req$53$1$2$2$1$0$1$0$0$1$#bcm_cpwr_cmd$12$1$2$2$1$0$1$0$0$1$#bcm_cpwr_mon$13$1$2$2$1$0$1$0$0$1$#bcm_epo$1$1$2$2$1$0$1$0$0$1$#bcm_gfd$16$12$2$2$1$0$2.500000e-01$0$0$1000$#bcm_hvil_mon$3$1$2$2$1$0$1$0$0$1$#bcm_ibat$40$16$2$2$1$0$2.500000e-02$-1000$-1000$500$#bcm_lls_status$54$2$2$2$1$0$1$0$0$3$#bcm_mainc_stat$4$2$2$2$1$0$1$0$0$2$#bcm_on_plug$2$1$2$2$1$0$1$0$0$1$#bcm_ready$0$1$2$2$1$0$1$0$0$1$#bcm_soc$24$8$2$2$1$0$5.000000e-01$0$0$100$#bcm_vbat$56$12$2$2$1$0$2.500000e-01$0$0$1000$#  NSignals=16  IDPort=off  TimestampPort=off  ErrorPort=off  RemotePort=off  LengthPort=off  StatusPort=off  StartBits=str2num('[int32(14);int32(52);int32(6);int32(53);int32(12);int32(13);int32(1);int32(16);int32(3);int32(40);int32(54);int32(4);int32(2);int32(0);int32(24);int32(56)]')  SignalSizes=str2num('[int32(2);int32(1);int32(2);int32(1);int32(1);int32(1);int32(1);int32(12);int32(1);int32(16);int32(2);int32(2);int32(1);int32(1);int32(8);int32(12)]')  ByteOrders=str2num('[int32(2);int32(2);int32(2);int32(2);int32(2);int32(2);int32(2);int32(2);int32(2);int32(2);int32(2);int32(2);int32(2);int32(2);int32(2);int32(2)]')  DataTypes=str2num('[int32(2);int32(2);int32(2);int32(2);int32(2);int32(2);int32(2);int32(2);int32(2);int32(2);int32(2);int32(2);int32(2);int32(2);int32(2);int32(2)]')  MultiplexTypes=str2num('[int32(1);int32(1);int32(1);int32(1);int32(1);int32(1);int32(1);int32(1);int32(1);int32(1);int32(1);int32(1);int32(1);int32(1);int32(1);int32(1)]')  MultiplexValues=str2num('[double(0);double(0);double(0);double(0);double(0);double(0);double(0);double(0);double(0);double(0);double(0);double(0);double(0);double(0);double(0);double(0)]')  Factors=str2num('[double(1);double(1);double(1);double(1);double(1);double(1);double(1);double(2.500000e-01);double(1);double(2.500000e-02);double(1);double(1);double(1);double(1);double(5.000000e-01);double(2.500000e-01)]')  Offsets=str2num('[double(0);double(0);double(0);double(0);double(0);double(0);double(0);double(0);double(0);double(-1000);double(0);double(0);double(0);double(0);double(0);double(0)]')  Minimums=str2num('[double(0);double(0);double(0);double(0);double(0);double(0);double(0);double(0);double(0);double(-1000);double(0);double(0);double(0);double(0);double(0);double(0)]')  Maximums=str2num('[double(3);double(1);double(2);double(1);double(1);double(1);double(1);double(1000);double(1);double(500);double(3);double(2);double(1);double(1);double(100);double(1000)]')
      settings: DataFormat=CANdb specified signals
  CAN Unpack6 : canmsglib/CAN Unpack  CANdbFile=C:\Users\EcoCAR_HIL\Documents\Khanna\EcoSIM3_P1_0_PHEV_TCU\Final_DBC\BCM_VehBus_Std.dbc  MsgList=BCM_Data1  MsgName=BCM_Data1  MsgIDType=Standard (11-bit identifier)  MsgIdentifier=1072  MsgLength=8  SignalInfo=bcm_cell_tmax$32$8$2$2$1$0$5.000000e-01$-40$-40$85$#bcm_cell_tmin$40$8$2$2$1$0$5.000000e-01$-40$-40$85$#bcm_cell_vmax$8$13$2$2$1$0$1.000000e-03$0$0$5$#bcm_cell_vmin$24$13$2$2$1$0$1.000000e-03$0$0$5$#bcm_chga_ena$7$1$2$2$1$0$1$0$0$1$#bcm_chga_mon$22$1$2$2$1$0$1$0$0$1$#bcm_lvbat$56$8$2$2$1$0$1.000000e-01$0$0$25$#bcm_mod_ena$23$1$2$2$1$0$1$0$0$1$#bcm_veh_mon$21$1$2$2$1$0$1$0$0$1$#  NSignals=9  IDPort=off  TimestampPort=off  ErrorPort=off  RemotePort=off  LengthPort=off  StatusPort=off  StartBits=str2num('[int32(32);int32(40);int32(8);int32(24);int32(7);int32(22);int32(56);int32(23);int32(21)]')  SignalSizes=str2num('[int32(8);int32(8);int32(13);int32(13);int32(1);int32(1);int32(8);int32(1);int32(1)]')  ByteOrders=str2num('[int32(2);int32(2);int32(2);int32(2);int32(2);int32(2);int32(2);int32(2);int32(2)]')  DataTypes=str2num('[int32(2);int32(2);int32(2);int32(2);int32(2);int32(2);int32(2);int32(2);int32(2)]')  MultiplexTypes=str2num('[int32(1);int32(1);int32(1);int32(1);int32(1);int32(1);int32(1);int32(1);int32(1)]')  MultiplexValues=str2num('[double(0);double(0);double(0);double(0);double(0);double(0);double(0);double(0);double(0)]')  Factors=str2num('[double(5.000000e-01);double(5.000000e-01);double(1.000000e-03);double(1.000000e-03);double(1);double(1);double(1.000000e-01);double(1);double(1)]')  Offsets=str2num('[double(-40);double(-40);double(0);double(0);double(0);double(0);double(0);double(0);double(0)]')  Minimums=str2num('[double(-40);double(-40);double(0);double(0);double(0);double(0);double(0);double(0);double(0)]')  Maximums=str2num('[double(85);double(85);double(5);double(5);double(1);double(1);double(25);double(1);double(1)]')
      settings: DataFormat=CANdb specified signals
  Scope : Scope
      settings: SaveName=ScopeData10
  Terminator{1..8,33..38} (14 alike) : Terminator
  Terminator_{15..19} (5 alike) : Terminator
  ESSTransmit : Outport
  wires:
  CAN Receive2/1 -> Terminator2/1
  Bus Creator2/1 -> ESSTransmit/1  "ESS_CAN_Out"
  CAN Unpack2/1 -> Terminator3/1
  CAN Unpack2/2 -> Terminator4/1
  CAN Unpack2/4 -> Terminator5/1
  CAN Unpack2/8 -> Terminator6/1
  CAN Unpack2/11 -> Terminator8/1
  CAN Unpack2/13 -> Bus Creator1/8  "bcm_on_plug"
  CAN Unpack6/1 -> Bus Creator/1  "bcm_cell_tmax"
  CAN Unpack6/2 -> Bus Creator/2  "bcm_cell_tmin"
  CAN Unpack6/3 -> Terminator33/1
  CAN Unpack6/4 -> Terminator34/1
  CAN Unpack6/5 -> Terminator35/1
  CAN Unpack6/6 -> Terminator36/1
  CAN Unpack6/7 -> Terminator37/1
  CAN Unpack6/8 -> Terminator38/1
  CAN Unpack6/9 -> Bus Creator/3  "bcm_veh_mon"
  CAN Unpack2/3 -> Bus Creator1/1  "bcm_chgc_stat"
  CAN Unpack2/5 -> Bus Creator1/2  "bcm_cpwr_cmd"
  CAN Unpack2/6 -> Bus Creator1/3  "bcm_cpwr_mon"
  CAN Unpack2/7 -> Bus Creator1/4  "bcm_epo"
  CAN Unpack2/9 -> Bus Creator1/5  "bcm_hvil_mon"
  CAN Unpack2/10 -> Bus Creator1/6  "bcm_ibat"
  CAN Unpack2/12 -> Scope/1, Bus Creator1/7  "bcm_mainc_stat"
  CAN Unpack2/14 -> Bus Creator1/9  "bcm_ready"
  CAN Unpack2/15 -> Bus Creator1/10  "bcm_soc"
  CAN Unpack2/16 -> Bus Creator1/11  "bcm_vbat"
  CAN Unpack1/3 -> Bus Creator3/1
  CAN Unpack1/5 -> Bus Creator3/2
  Bus Creator1/1 -> Bus Creator2/1  "BCM_Status"
  Bus Creator/1 -> Bus Creator2/2  "BCM_Data1"
  Bus Creator3/1 -> Bus Creator2/3  "BCM_Limits"
  CAN Unpack1/1 -> Terminator_15/1
  CAN Unpack1/2 -> Terminator_16/1
  CAN Unpack1/4 -> Terminator_17/1
  CAN Unpack1/6 -> Terminator_18/1
  CAN Unpack1/7 -> Terminator_19/1
  CAN Receive1/1 -> Terminator1/1
  CAN Receive3/1 -> Terminator7/1
  CAN Receive2/2 -> CAN Unpack2/1
  CAN Receive1/2 -> CAN Unpack6/1
  CAN Receive3/2 -> CAN Unpack1/1
